simulink model "OrbitPropagatorBlockExampleModel"  (R2022a)
settings: Solver=VariableStepAuto  StartTime=0.0  StopTime=86400  FixedStep=5  MinStep=10  RelTol=1e-6  AbsTol=1e-7
model workspace (MATLAB code in the model file):
  | initialize6DOFSkyHogg;
settings Model: Creator=The MathWorks, Inc.  LastModifiedBy=fernanda
settings SolverCC: MaxConsecutiveMinStep=5  AlgebraicLoopSolver=TrustRegion  AutoInsertRateTranBlk=on  InsertRTBMode=Never (minimum delay)  MinimalZcImpactIntegration=on
settings DataIOCC: SignalLogging=off  DSMLogging=off  SaveTime=off
settings OptimizationCC: EnhancedBackFolding=on  StrengthReduction=on  InitFltsAndDblsToZero=on  DifferentSizesBufferReuse=on
settings DebuggingCC: WriteAfterWriteMsg=DisableAll  AlgebraicLoopMsg=none  FcnCallInpInsideContextMsg=warning  UniqueDataStoreMsg=error  RootOutportRequireBusObject=none  StateNameClashWarn=warning  PregeneratedLibrarySubsystemCodeDiagnostic=none  StrictBusMsg=ErrorOnBusTreatedAsVector  SFUnexpectedBacktrackingDiag=warning  SFNoUnconditionalDefaultTransitionDiag=warning  SFExecutionAtInitializationDiag=none  SFMachineParentedDataDiag=warning  ArithmeticOperatorsInVariantConditions=warning
settings ModelReferenceCC: PropagateSignalLabelsOutOfModel=off
settings SFSimCC: SimUseLocalCustomCode=off
settings RTWCC: RTWUseLocalCustomCode=off  DLArmComputeVersion=19.05
settings CodeAppCC: StateflowObjectComments=on

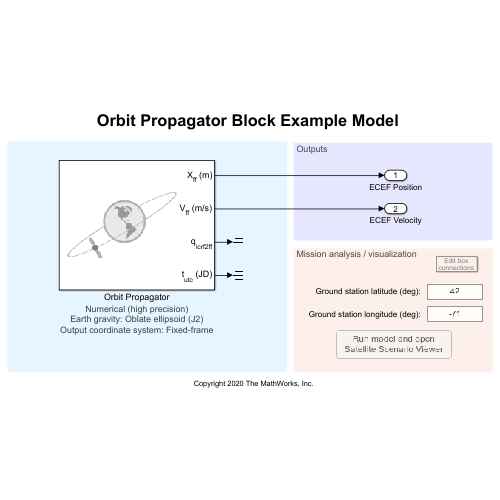
[thumbnail: Simulink's stored preview of the top-level diagram]
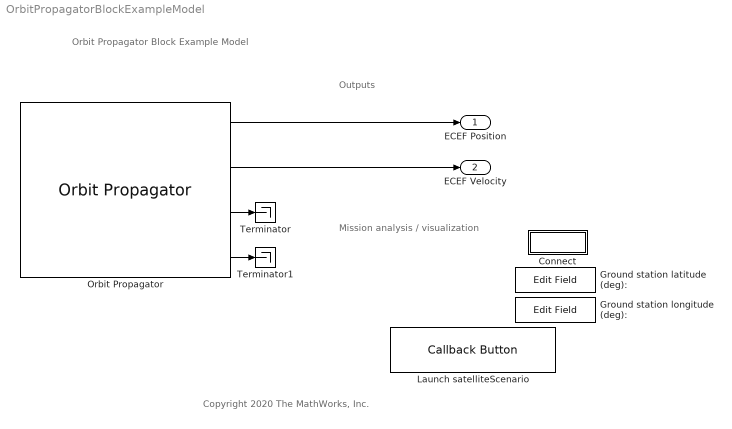
== system OrbitPropagatorBlockExampleModel ==
  note: Copyright 2020 The MathWorks, Inc.
  note: Orbit Propagator Block Example Model
  note: Mission analysis / visualization
  note: Outputs
  Connect : Subsystem
      mask Display: disp("Edit box\nconnections")
  Ground station latitude (deg): : EditField  LabelPosition=Hide  ShowInitialText=on  Alignment=Center
  Ground station longitude (deg): : EditField  LabelPosition=Hide  ShowInitialText=on  Alignment=Center
  Launch satelliteScenario : CallbackButton  ButtonText=Run model and open Satellite Scenario Viewer
      settings: ClickFcn=|
      | % Find orbit propagator block in model
      | cb.mdl = bdroot(gcb);
      | cb.blk = Simulink.findBlocksOfType(cb.mdl,"OrbitPropagator");
      | 
      | % Create Simulation input object to run model
      | cb.simInput = Simulink.SimulationInput(cb.mdl);
      | cb.simInput = setModelParameter(cb.simInput, ...
      |     "SolverType", "Variable-step", "SolverName", "VariableStepAuto", ...
      |     "RelTol", "1e-7", "AbsTol", "1e-8", ...
      |     "SaveOutput", "on", "OutputSaveName", "yout", ...
      |     "SaveFormat", "Dataset");
      | 
      | % Run the model
      | cb.out = sim(cb.simInput);
      | 
      | % Extract timeseries data from Simulation output object
      | cb.timeseriesPosECEF = cb.out.yout{1}.Values;
      | cb.timeseriesPosECEF.TimeInfo.StartDate = ...
      |     datetime(eval(get_param(cb.blk,'startDate')), "convertFrom", "juliandate");
      | cb.timeseriesVelECEF = cb.out.yout{2}.Values;
      | 
      | % Create satellite scenario
      | scenario_OrbitPropExample = satelliteScenario;
      | 
      | % Add satellites from timeseries data
      | cb.tsSize = size(cb.timeseriesPosECEF.Data);
      | cb.numSats = cb.tsSize(cb.tsSize ~= cb.timeseriesPosECEF.Length & cb.tsSize ~= 3);
      | if isempty(cb.numSats); cb.numSats = 3; end
      | cb.names = "Satellite " + (1:cb.numSats);
      | cb.sat = satellite(scenario_OrbitPropExample, cb.timeseriesPosECEF, cb.timeseriesVelECEF, ...
      |     "CoordinateFrame", "ecef", "Name", cb.names);
      | 
      | % Set satellite graphical properties
      | cb.colorMap = lines(256); cb.colorMap(1:3, :) = [];
      | for cbidx = 1:numel(cb.sat)
      |     cb.sat(cbidx).Orbit.LineColor = cb.colorMap(cbidx,:);
      |     cb.sat(cbidx).MarkerColor = cb.colorMap(cbidx,:);
      |     cb.sat(cbidx).LabelFontColor = cb.colorMap(cbidx,:);
      |     cb.sat(cbidx).GroundTrack.LeadLineColor = cb.colorMap(cbidx,:);
      | end
      | 
      | % Add ground station to scenario
      | cb.gs = groundStation(scenario_OrbitPropExample, str2double(get_param(cb.mdl+"/Connect/LatVal", "Value")),...
      |    str2double(get_param(cb.mdl+"/Connect/LonVal", "Value")), "MinElevationAngle", 10, ...
      |    "Name", "Ground Station");
      | 
      | % Add access analysis between each satellite and the ground station
      | for cbidx = 1:numel(cb.sat)
      |     cb.ac(cbidx) = access(cb.sat(cbidx), cb.gs);
      |     cb.ac(cbidx).LineColor = "green";
      | end
      | 
      | % Clean up variables created in base workspace
      | clear cb cbidx;
      | 
      | % Open and animate scenario
      | play(scenario_OrbitPropExample);
      | 
      | % Scenario object scenario_OrbitPropExample is in the base workspace for further analysis
  Orbit Propagator : OrbitPropagator  propagator=Numerical (high precision)  outportFrame=Fixed-frame  startDate=2459730.4329  semiMajorAxis=mission.Satellites.SemiMajorAxis  eccentricity=mission.Satellites.Eccentricity  inclination=mission.Satellites.Inclination  raan=mission.Satellites.RAAN  argPeriapsis=mission.Satellites.ArgOfPeriapsis  trueAnomaly=mission.Satellites.TrueAnomaly  inertialPosition=[3649700.0 3308200.0 -4676600.0]  inertialVelocity=[-2750.8 6666.4 2573.4]  fixedPosition=[-4142689.0 -2676864.7 -4669861.6]  fixedVelocity=[1452.7 -6720.7 2568.1]  gravityModel=Oblate ellipsoid (J2)  customR=3396200  customMu=4.305e13  customJ2=1.0826269e-03  customOmega=4.06125949e-3  useEOPs=off  outputTransform=on
      settings: AttributesFormatString=|
      | %<propagator>
      | Earth gravity: %<gravityModel>
      | Output coordinate system: %<outportFrame>
  Terminator : Terminator
  Terminator1 : Terminator
  ECEF Position : Outport
  ECEF Velocity : Outport  Port=2
  wires:
  Orbit Propagator/4 -> Terminator1/1
  Orbit Propagator/3 -> Terminator/1
  Orbit Propagator/1 -> ECEF Position/1
  Orbit Propagator/2 -> ECEF Velocity/1

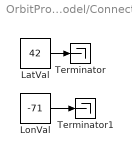
== system OrbitPropagatorBlockExampleModel/Connect ==
  LatVal : Constant  Value=42
  LonVal : Constant  Value=-71
  Terminator : Terminator
  Terminator1 : Terminator
  wires:
  LatVal/1 -> Terminator/1
  LonVal/1 -> Terminator1/1
